simulink model "r4_pfb_fir"  (Simulink 7.0)
settings: Solver=FixedStepDiscrete  SolverMode=SingleTasking  StartTime=0.0  StopTime=10.0  RelTol=1e-3
undefined symbols (not defined in the file): pfb_coefs
libraries: xbsIndex_r4 x385, xps_library x1
(part 27 of 27)

== system r4_pfb_fir/fir_2/fir_tap_6/fir_coef/c_gen ==
  sync_in : Inport  OutDataType=sfix(16)  OutScaling=2^0
  Counter : xbsIndex_r4/Counter  cnt_type=Count Limited  cnt_to=1023  operation=Up  start_count=0  cnt_by_val=1  arith_type=Unsigned  n_bits=10  bin_pt=0  load_pin=off  rst=on  en=off  explicit_period=off  period=1  dbl_ovrd=off  use_behavioral_HDL=off  use_rpm=on  implementation=Fabric  block_type=counter
      settings: xl_area=[0, 0, 0, 0, 0, 0, 0]
  addr_sel : xbsIndex_r4/Slice  nbits=10  boolean_output=off  mode=Upper Bit Location + Width  bit1=0  base1=MSB of Input  bit0=-1  base0=MSB of Input  dbl_ovrd=off  block_type=slice
      settings: infoedit="Extracts a given range of bits from each input sample and presents it at the output.  The output type is ordinarily unsigned with binary point at zero, but can be Boolean when the slice is one bit wide.<P><P>Hardware notes: In hardware this block costs nothing."  block_version=10.1.3
  mem : xbsIndex_r4/ROM  depth=1024  initVector=[0;0;0;0;0;0;0;0;0;0;0;0;0;0;0;0;0;0;0;0;0;0;0;0;0;0;0;0;0;0;0;0;0;0;0;0;0;0;0;0;0;0;0;0;0;0;0;0;0;0;0;0;0;0;0;0;0;0;0;0;0;0;0;0;0;0;0;0;0;0;0;0;0;0.00390625;0.00390625;0.00390625;0.00390625;0.00390625;0.00390625;0.00390625;0.00390625;0.00390625;0.00390625;0.00390625;0.00390625;0.00390625;0.00390625;0.00390625;0.00390625;0.00390625;0.00390625;0.00390625;0.00390625;0.00390625;0.00390625;0.00390625;0.00390625;0.00390625;0.00390625;0.00390625;0.00390625;0.00390625;0.00390625;0.00390625;0.00390625;0.00390625;0.00390625;0.00390625;0.00390625;0.00390625;0.00390625;0.00390625;0.00390625;0.00390625;0.00390625;0.00390625;0.00390625;0.00390625;0.00390625;0.00390625;0.00390625;0.00390625;0.00390625;0.00390625;0.00390625;0.00390625;0.00390625;0.00390625;0.00390625;0.00390625;0.00390625;0.00390625;0.00390625;0.00390625;0.00390625;0.00390625;0.00390625;0.00390625;0.00390625;0.00390625;0.00390625;0.00390625;0.00390625;0.00390625;0.00390625;0.00390625;0.00390625;0.00390625;0.00390625;0.00390625;0.00390625;0.00390625;0.00390625;0.00390625;0.00390625;0.00390625;0.00390625;0.00390625;0.00390625;0.00390625;0.00390625;0.00390625;0.00390625;0.00390625;0.00390625;0.00390625;0.00390625;0.00390625;0.00390625;0.00390625;0.00390625;0.00390625;0.00390625;0.00390625;0.00390625;0.00390625;0.00390625;0.00390625;0.00390625;0.00390625;0.00390625;0.00390625;0.00390625;0.00390625;0.00390625;0.00390625;0.00390625;0.00390625;0.00390625;0.00390625;0.00390625;0.00390625;0.00390625;0.00390625;0.00390625;0.00390625;0.00390625;0.00390625;0.00390625;0.00390625;0.0078125;0.0078125;0.0078125;0.0078125;0.0078125;0.0078125;0.0078125;0.0078125;0.0078125;0.0078125;0.0078125;0.0078125;0.0078125;0.0078125;0.0078125;0.0078125;0.0078125;0.0078125;0.0078125;0.0078125;0.0078125;0.0078125;0.0078125;0.0078125;0.0078125;0.0078125;0.0078125;0.0078125;0.0078125;0.0078125;0.0078125;0.0078125;0.0078125;0.0078125;0.0078125;0.0078125;0.0078125;0.0078125;0.0078125;0.0078125;0.0078125;0.0078125;0.0078125;0.0078125;0.0078125;0.0078125;0.0078125;0.0078125;0.0078125;0.0078125;0.0078125;0.0078125;0.0078125;0.0078125;0.0078125;0.0078125;0.0078125;0.0078125;0.0078125;0.0078125;0.0078125;0.0078125;0.0078125;0.0078125;0.0078125;0.0078125;0.0078125;0.0078125;0.0078125;0.0078125;0.0078125;0.0078125;0.0078125;0.0078125;0.0078125;0.0078125;0.0078125;0.0078125;0.0078125;0.0078125;0.0078125;0.0078125;0.0078125;0.0078125;0.0078125;0.0078125;0.0078125;0.0078125;0.0078125;0.0078125;0.0078125;0.0078125;0.0078125;0.0078125;0.0078125;0.0078125;0.0078125;0.0078125;0.0078125;0.0078125;0.0078125;0.0078125;0.0078125;0.0078125;0.0078125;0.0078125;0.0078125;0.01171875;0.01171875;0.01171875;0.01171875;0.01171875;0.01171875;0.01171875;0.01171875;0.01171875;0.01171875;0.01171875;0.01171875;0.01171875;0.01171875;0.01171875;0.01171875;0.01171875;0.01171875;0.01171875;0.01171875;0.01171875;0.01171875;0.01171875;0.01171875;0.01171875;0.01171875;0.01171875;0.01171875;0.01171875;0.01171875;0.01171875;0.01171875;0.01171875;0.01171875;0.01171875;0.01171875;0.01171875;0.01171875;0.01171875;0.01171875;0.01171875;0.01171875;0.01171875;0.01171875;0.01171875;0.01171875;0.01171875;0.01171875;0.01171875;0.01171875;0.01171875;0.01171875;0.01171875;0.01171875;0.01171875;0.01171875;0.01171875;0.01171875;0.01171875;0.01171875;0.01171875;0.01171875;0.01171875;0.01171875;0.01171875;0.01171875;0.01171875;0.01171875;0.01171875;0.01171875;0.01171875;0.01171875;0.01171875;0.01171875;0.01171875;0.01171875;0.01171875;0.01171875;0.01171875;0.01171875;0.01171875;0.01171875;0.01171875;0.01171875;0.01171875;0.01171875;0.01171875;0.01171875;0.01171875;0.01171875;0.01171875;0.01171875;0.01171875;0.01171875;0.01171875;0.01171875;0.015625;0.015625;0.015625;0.015625;0.015625;0.015625;0.015625;0.015625;0.015625;0.015625;0.015625;0.015625;0.015625;0.015625;0.015625;0.015625;0.015625;0.015625;0.015625;0.015625;0.015625;0.015625;0.015625;0.015625;0.015625;0.015625;0.015625;0.015625;0.015625;0.015625;0.015625;0.015625;0.015625;0.015625;0.015625;0.015625 ...(+5924 chars)]  distributed_mem=Block RAM  rst=off  init_reg=0  en=off  latency=1  arith_type="Signed  (2's comp)"  n_bits=9  bin_pt=8  dbl_ovrd=off  optimize=Area  use_rpm=on  block_type=sprom
      settings: AttributesFormatString=depth = %<depth>\ndist_mem = %<distributed_mem>  xl_area=[0, 0, 0, 0, 0, 0, 0]  block_version=10.1.3
  coef_out : Outport  OutDataType=sfix(16)  OutScaling=2^0
  wires:
  sync_in/1 -> Counter/1
  Counter/1 -> addr_sel/1
  addr_sel/1 -> mem/1
  mem/1 -> coef_out/1

== system r4_pfb_fir/fir_2/fir_tap_6/fir_core/c_to_ri_d ==
  c : Inport  OutDataType=sfix(16)  OutScaling=2^0
  force_im : xbsIndex_r4/Reinterpret  force_arith_type=on  arith_type="Signed  (2's comp)"  force_bin_pt=on  bin_pt=7  block_type=reinterpret
      settings: infoedit="Changes signal type without altering the binary representation.   You can changed the signal between signed and unsigned, and relocate the binary point.<P><P>Hardware notes: In hardware this block costs nothing.<P><P>Example:  Suppose the input is 6 bits wide, signed, with 2 fractional bits, and the output is forced to unsigned with 0 fractional bits.  Then an input of -2.0 (1110.00 in binary 2's complement) becomes an output of 56 (111000 in binary)."  block_version=10.1.3
  force_re : xbsIndex_r4/Reinterpret  force_arith_type=on  arith_type="Signed  (2's comp)"  force_bin_pt=on  bin_pt=7  block_type=reinterpret
      settings: infoedit="Changes signal type without altering the binary representation.   You can changed the signal between signed and unsigned, and relocate the binary point.<P><P>Hardware notes: In hardware this block costs nothing.<P><P>Example:  Suppose the input is 6 bits wide, signed, with 2 fractional bits, and the output is forced to unsigned with 0 fractional bits.  Then an input of -2.0 (1110.00 in binary 2's complement) becomes an output of 56 (111000 in binary)."  block_version=10.1.3
  slice_im : xbsIndex_r4/Slice  nbits=8  boolean_output=off  mode=Lower Bit Location + Width  bit1=0  base1=MSB of Input  bit0=0  base0=LSB of Input  dbl_ovrd=off  block_type=slice
      settings: infoedit="Extracts a given range of bits from each input sample and presents it at the output.  The output type is ordinarily unsigned with binary point at zero, but can be Boolean when the slice is one bit wide.<P><P>Hardware notes: In hardware this block costs nothing."  block_version=10.1.3
  slice_re : xbsIndex_r4/Slice  nbits=8  boolean_output=off  mode=Upper Bit Location + Width  bit1=0  base1=MSB of Input  bit0=0  base0=LSB of Input  dbl_ovrd=off  block_type=slice
      settings: infoedit="Extracts a given range of bits from each input sample and presents it at the output.  The output type is ordinarily unsigned with binary point at zero, but can be Boolean when the slice is one bit wide.<P><P>Hardware notes: In hardware this block costs nothing."  block_version=10.1.3
  re : Outport  OutDataType=sfix(16)  OutScaling=2^0
  im : Outport  Port=2  OutDataType=sfix(16)  OutScaling=2^0
  wires:
  slice_re/1 -> force_re/1
  slice_im/1 -> force_im/1
  force_re/1 -> re/1
  force_im/1 -> im/1
  c/1 -> slice_re/1, slice_im/1

== system r4_pfb_fir/fir_2/fir_tap_6/fir_core/c_to_ri_s ==
  c : Inport  OutDataType=sfix(16)  OutScaling=2^0
  force_im : xbsIndex_r4/Reinterpret  force_arith_type=on  arith_type="Signed  (2's comp)"  force_bin_pt=on  bin_pt=15  block_type=reinterpret
      settings: infoedit="Changes signal type without altering the binary representation.   You can changed the signal between signed and unsigned, and relocate the binary point.<P><P>Hardware notes: In hardware this block costs nothing.<P><P>Example:  Suppose the input is 6 bits wide, signed, with 2 fractional bits, and the output is forced to unsigned with 0 fractional bits.  Then an input of -2.0 (1110.00 in binary 2's complement) becomes an output of 56 (111000 in binary)."  block_version=10.1.3
  force_re : xbsIndex_r4/Reinterpret  force_arith_type=on  arith_type="Signed  (2's comp)"  force_bin_pt=on  bin_pt=15  block_type=reinterpret
      settings: infoedit="Changes signal type without altering the binary representation.   You can changed the signal between signed and unsigned, and relocate the binary point.<P><P>Hardware notes: In hardware this block costs nothing.<P><P>Example:  Suppose the input is 6 bits wide, signed, with 2 fractional bits, and the output is forced to unsigned with 0 fractional bits.  Then an input of -2.0 (1110.00 in binary 2's complement) becomes an output of 56 (111000 in binary)."  block_version=10.1.3
  slice_im : xbsIndex_r4/Slice  nbits=17  boolean_output=off  mode=Lower Bit Location + Width  bit1=0  base1=MSB of Input  bit0=0  base0=LSB of Input  dbl_ovrd=off  block_type=slice
      settings: infoedit="Extracts a given range of bits from each input sample and presents it at the output.  The output type is ordinarily unsigned with binary point at zero, but can be Boolean when the slice is one bit wide.<P><P>Hardware notes: In hardware this block costs nothing."  block_version=10.1.3
  slice_re : xbsIndex_r4/Slice  nbits=17  boolean_output=off  mode=Upper Bit Location + Width  bit1=0  base1=MSB of Input  bit0=0  base0=LSB of Input  dbl_ovrd=off  block_type=slice
      settings: infoedit="Extracts a given range of bits from each input sample and presents it at the output.  The output type is ordinarily unsigned with binary point at zero, but can be Boolean when the slice is one bit wide.<P><P>Hardware notes: In hardware this block costs nothing."  block_version=10.1.3
  re : Outport  OutDataType=sfix(16)  OutScaling=2^0
  im : Outport  Port=2  OutDataType=sfix(16)  OutScaling=2^0
  wires:
  slice_re/1 -> force_re/1
  slice_im/1 -> force_im/1
  force_re/1 -> re/1
  force_im/1 -> im/1
  c/1 -> slice_re/1, slice_im/1

== system r4_pfb_fir/fir_2/fir_tap_6/fir_core/mult_add_im ==
  a : Inport  OutDataType=sfix(16)  OutScaling=2^0
  b : Inport  Port=2  OutDataType=sfix(16)  OutScaling=2^0
  c : Inport  Port=3  OutDataType=sfix(16)  OutScaling=2^0
  add : xbsIndex_r4/AddSub  mode=Addition  use_carryin=off  use_carryout=off  en=off  latency=1  precision=Full  arith_type="Signed  (2's comp)"  n_bits=9  bin_pt=7  quantization=Truncate  overflow=Wrap  dbl_ovrd=off  use_behavioral_HDL=on  pipelined=on  use_rpm=on  hw_selection=Fabric  block_type=addsub
      settings: xl_area=[0, 0, 0, 0, 0, 0, 0]  block_version=10.1.3
  delay : xbsIndex_r4/Delay  en=off  latency=3  dbl_ovrd=off  reg_retiming=off  block_type=delay
      settings: xl_area=[0, 0, 0, 0, 0, 0, 0]
  mult : xbsIndex_r4/Mult  precision=Full  arith_type="Signed  (2's comp)"  n_bits=8  bin_pt=2  quantization=Truncate  overflow=Wrap  en=off  latency=3  dbl_ovrd=off  use_behavioral_HDL=off  use_embedded=on  opt=Speed  optimum_pipeline=off  pipeline=on  use_rpm=on  placement_style=Rectangular shape  block_type=mult
      settings: infoedit=Hardware notes: To use the internal pipeline stage of the dedicated multiplier you must select 'Pipeline for maximum performance'.  xl_area=[0, 0, 0, 0, 0, 0, 0]  block_version=10.1.3
  out : Outport  OutDataType=sfix(16)  OutScaling=2^0
  wires:
  add/1 -> out/1
  mult/1 -> add/1
  delay/1 -> add/2
  a/1 -> mult/1
  b/1 -> mult/2
  c/1 -> delay/1

== system r4_pfb_fir/fir_2/fir_tap_6/fir_core/mult_add_re ==
  a : Inport  OutDataType=sfix(16)  OutScaling=2^0
  b : Inport  Port=2  OutDataType=sfix(16)  OutScaling=2^0
  c : Inport  Port=3  OutDataType=sfix(16)  OutScaling=2^0
  add : xbsIndex_r4/AddSub  mode=Addition  use_carryin=off  use_carryout=off  en=off  latency=1  precision=Full  arith_type="Signed  (2's comp)"  n_bits=9  bin_pt=7  quantization=Truncate  overflow=Wrap  dbl_ovrd=off  use_behavioral_HDL=on  pipelined=on  use_rpm=on  hw_selection=Fabric  block_type=addsub
      settings: xl_area=[0, 0, 0, 0, 0, 0, 0]  block_version=10.1.3
  delay : xbsIndex_r4/Delay  en=off  latency=3  dbl_ovrd=off  reg_retiming=off  block_type=delay
      settings: xl_area=[0, 0, 0, 0, 0, 0, 0]
  mult : xbsIndex_r4/Mult  precision=Full  arith_type="Signed  (2's comp)"  n_bits=8  bin_pt=2  quantization=Truncate  overflow=Wrap  en=off  latency=3  dbl_ovrd=off  use_behavioral_HDL=off  use_embedded=on  opt=Speed  optimum_pipeline=off  pipeline=on  use_rpm=on  placement_style=Rectangular shape  block_type=mult
      settings: infoedit=Hardware notes: To use the internal pipeline stage of the dedicated multiplier you must select 'Pipeline for maximum performance'.  xl_area=[0, 0, 0, 0, 0, 0, 0]  block_version=10.1.3
  out : Outport  OutDataType=sfix(16)  OutScaling=2^0
  wires:
  add/1 -> out/1
  mult/1 -> add/1
  delay/1 -> add/2
  a/1 -> mult/1
  b/1 -> mult/2
  c/1 -> delay/1

== system r4_pfb_fir/fir_2/fir_tap_6/fir_core/ri_to_c ==
  re : Inport  OutDataType=sfix(16)  OutScaling=2^0
  im : Inport  Port=2  OutDataType=sfix(16)  OutScaling=2^0
  concat : xbsIndex_r4/Concat  num_inputs=2  dbl_ovrd=off  block_type=concat
      settings: block_version=10.1.3
  force_im : xbsIndex_r4/Reinterpret  force_arith_type=on  arith_type=Unsigned  force_bin_pt=on  bin_pt=0  block_type=reinterpret
      settings: infoedit="Changes signal type without altering the binary representation.   You can changed the signal between signed and unsigned, and relocate the binary point.<P><P>Hardware notes: In hardware this block costs nothing.<P><P>Example:  Suppose the input is 6 bits wide, signed, with 2 fractional bits, and the output is forced to unsigned with 0 fractional bits.  Then an input of -2.0 (1110.00 in binary 2's complement) becomes an output of 56 (111000 in binary)."  block_version=10.1.3
  force_re : xbsIndex_r4/Reinterpret  force_arith_type=on  arith_type=Unsigned  force_bin_pt=on  bin_pt=0  block_type=reinterpret
      settings: infoedit="Changes signal type without altering the binary representation.   You can changed the signal between signed and unsigned, and relocate the binary point.<P><P>Hardware notes: In hardware this block costs nothing.<P><P>Example:  Suppose the input is 6 bits wide, signed, with 2 fractional bits, and the output is forced to unsigned with 0 fractional bits.  Then an input of -2.0 (1110.00 in binary 2's complement) becomes an output of 56 (111000 in binary)."  block_version=10.1.3
  c : Outport  OutDataType=sfix(16)  OutScaling=2^0
  wires:
  im/1 -> force_im/1
  concat/1 -> c/1
  re/1 -> force_re/1
  force_im/1 -> concat/2
  force_re/1 -> concat/1

== system r4_pfb_fir/fir_2/fir_tap_6/fir_core/tap_delay ==
  in : Inport  OutDataType=sfix(16)  OutScaling=2^0
  slr : xbsIndex_r4/Delay  en=off  latency=0  dbl_ovrd=off  reg_retiming=off  block_type=delay
      settings: xl_area=[0, 0, 0, 0, 0, 0, 0]
  out : Outport  OutDataType=sfix(16)  OutScaling=2^0
  wires:
  slr/1 -> out/1
  in/1 -> slr/1
